simulink model "lab2_LPF"  (R2016b)
settings: Solver=VariableStepAuto  StartTime=0.0  StopTime=10.0  RelTol=1e-3
settings Model: Creator=MSI  LastModifiedBy=EE103
settings OptimizationCC: LifeSpan=inf
settings DebuggingCC: SFExecutionAtInitializationDiag=none
settings SFSimCC: SimUseLocalCustomCode=on
settings RTWCC: RTWUseLocalCustomCode=on

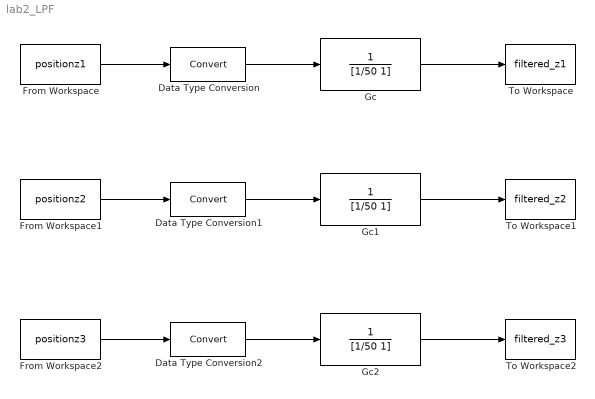
== system lab2_LPF ==
  Data Type Conversion : DataTypeConversion
  Data Type Conversion1 : DataTypeConversion
  Data Type Conversion2 : DataTypeConversion
  From Workspace : FromWorkspace  VariableName=positionz1  SampleTime=0.01
  From Workspace1 : FromWorkspace  VariableName=positionz2  SampleTime=0.01
  From Workspace2 : FromWorkspace  VariableName=positionz3  SampleTime=0.01
  Gc : TransferFcn  Numerator=1  Denominator=[1/50 1]
  Gc1 : TransferFcn  Numerator=1  Denominator=[1/50 1]
  Gc2 : TransferFcn  Numerator=1  Denominator=[1/50 1]
  To Workspace : ToWorkspace  VariableName=filtered_z1  SaveFormat=Timeseries  SampleTime=-1
  To Workspace1 : ToWorkspace  VariableName=filtered_z2  SaveFormat=Timeseries  SampleTime=-1
  To Workspace2 : ToWorkspace  VariableName=filtered_z3  SaveFormat=Timeseries  SampleTime=-1
  wires:
  From Workspace/1 -> Data Type Conversion/1
  Gc/1 -> To Workspace/1
  Data Type Conversion/1 -> Gc/1
  From Workspace1/1 -> Data Type Conversion1/1
  Gc1/1 -> To Workspace1/1
  Data Type Conversion1/1 -> Gc1/1
  From Workspace2/1 -> Data Type Conversion2/1
  Gc2/1 -> To Workspace2/1
  Data Type Conversion2/1 -> Gc2/1
